simulink model "simPIFuzzy"  (R2023b)
settings: Solver=FixedStepAuto  StartTime=0.0  StopTime=initValues(2)  FixedStep=initValues(1)  RelTol=1e-3
values from neighbouring files (symbols this model uses):
  initValues = initialize()    [comparision.m]    (also in initialize.m = [T, tsim, stepValue, upperLim, lowerLim, K, tau, pert]; programClassic.m; programFuzzy.m)
libraries: fuzblock x1
settings Model: Creator=usuario  LastModifiedBy=usuario
settings DataIOCC: ReturnWorkspaceOutputs=off

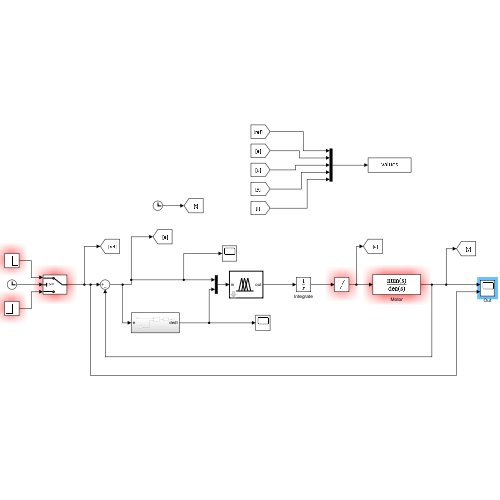
[thumbnail: Simulink's stored preview of the top-level diagram]
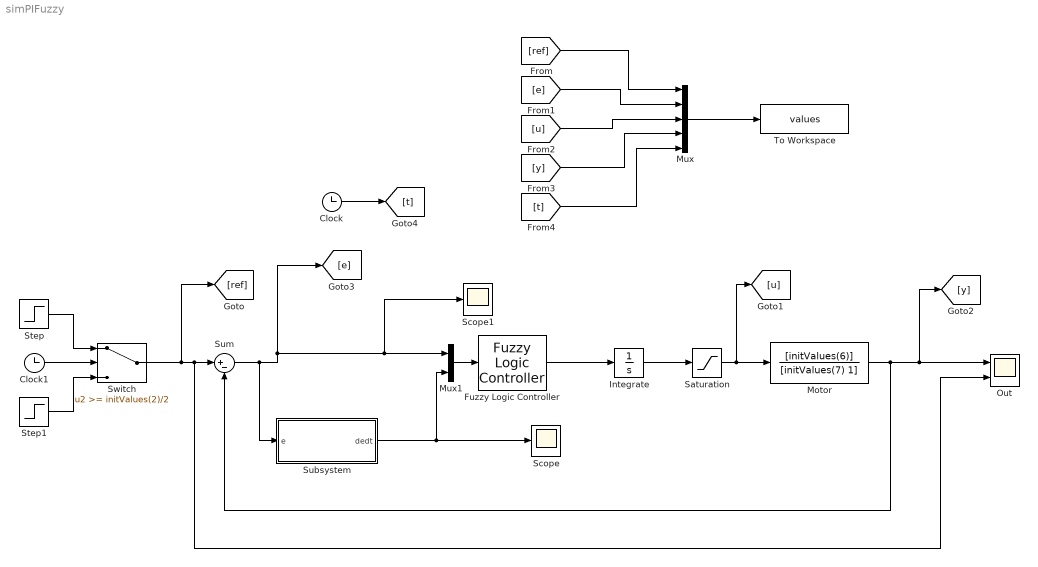
== system simPIFuzzy ==
  Clock : Clock
  Clock1 : Clock
  Fuzzy Logic Controller : fuzblock/Fuzzy Logic  Controller  FIS='fuzzyPI.fis'  OutputSampleNumber=101  DataType=double  FuzzifiedInputs=off  RuleFiringStrengths=off  RuleOutputs=off  AggregatedOutputs=off  SimulateUsing=Interpreted execution  OutOfRangeInputValueMessage=warning  NoRuleFiredMessage=warning  EmptyOutputFuzzySetMessage=warning
  Integrate : Integrator
  Motor : TransferFcn  Numerator=[initValues(6)]  Denominator=[initValues(7) 1]
  Mux : Mux  Inputs=5
  Mux1 : Mux  Inputs=2
  Out : Scope  NumInputPorts=2
  Saturation : Saturate  UpperLimit=initValues(4)  LowerLimit=initValues(5)
  Scope : Scope
  Scope1 : Scope
  Step : Step  After=-initValues(3)/2  SampleTime=0
  Step1 : Step  After=initValues(3)/2  SampleTime=0
  Subsystem : Subsystem
  Sum : Sum  Inputs=|+-
  Switch : Switch  Threshold=initValues(2)/2  SaturateOnIntegerOverflow=off  InputSameDT=off
  To Workspace : ToWorkspace  VariableName=values  SaveFormat=Structure  SampleTime=-1
  wires:
  Motor/1 -> Sum/2, [y], Out/1
  Switch/1 -> [ref], Out/2, Sum/1
  [ref] -> Mux/1
  [y] -> Mux/4
  [e] -> Mux/2
  [u] -> Mux/3
  Mux/1 -> To Workspace/1
  Saturation/1 -> [u], Motor/1
  Clock/1 -> [t]
  [t] -> Mux/5
  Clock1/1 -> Switch/2
  Step/1 -> Switch/1
  Step1/1 -> Switch/3
  Mux1/1 -> Fuzzy Logic Controller/1
  Sum/1 -> Subsystem/1(e), Scope1/1, Mux1/1, [e]
  Integrate/1 -> Saturation/1
  Fuzzy Logic Controller/1 -> Integrate/1
  Subsystem/1(dedt) -> Mux1/2, Scope/1

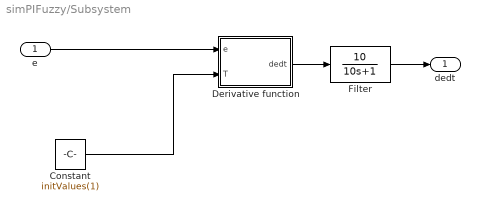
== system simPIFuzzy/Subsystem ==
  e : Inport
  Constant : Constant  Value=initValues(1)
  Derivative function : MATLAB Function  TreatAsAtomicUnit=on
  Filter : TransferFcn  Numerator=[10]  Denominator=[10 1]
  dedt : Outport
  wires:
  Constant/1 -> Derivative function/2(T)
  e/1 -> Derivative function/1(e)
  Derivative function/1(dedt) -> Filter/1
  Filter/1 -> dedt/1

== matlab function simPIFuzzy/Subsystem/Derivative function ==
  settings: updateMethod=DISCRETE  sampleTime=initValues(1)
  data: e input; dedt output; T input
function dedt = fcn(e, T)
    persistent pre_e;

    if isempty(pre_e)
        pre_e = e;
    end
    
    dedt = (pre_e - e)/T;
    pre_e = e;
end
